simulink model "D53_LKAS_JLU_20200909_1512"  (R2018b)
settings: Solver=ode3  StartTime=0.0  StopTime=10.0  FixedStep=0.01  RelTol=1e-3  EnableMultiTasking=on
model workspace (MAT data in the model file):
  MCOS : class17 (value not decoded)
  MCOS : class17 (value not decoded)
  MCOS : class17 (value not decoded)
  MCOS : class17 (value not decoded)
  MCOS : class17 (value not decoded)
  MCOS : class17 (value not decoded)
  MCOS : class17 (value not decoded)
  MCOS : class17 (value not decoded)
  MCOS : class17 (value not decoded)
  MCOS : class17 (value not decoded)
  MCOS : class17 (value not decoded)
  MCOS : class17 (value not decoded)
  MCOS : class17 (value not decoded)
  MCOS : class17 (value not decoded)
  MCOS : class17 (value not decoded)
  MCOS : class17 (value not decoded)
  MCOS : class17 (value not decoded)
  MCOS : class17 (value not decoded)
  MCOS : class17 (value not decoded)
  MCOS : class17 (value not decoded)
  MCOS : class17 (value not decoded)
  MCOS : class17 (value not decoded)
  MCOS : class17 (value not decoded)
  MCOS : class17 (value not decoded)
  MCOS : class17 (value not decoded)
  MCOS : class17 (value not decoded)
  MCOS : class17 (value not decoded)
  MCOS : class17 (value not decoded)
  MCOS : class17 (value not decoded)
  MCOS : class17 (value not decoded)
  MCOS : class17 (value not decoded)
  MCOS : class17 (value not decoded)
  MCOS : class17 (value not decoded)
  MCOS : class17 (value not decoded)
  MCOS : class17 (value not decoded)
  MCOS : class17 (value not decoded)
  MCOS : class17 (value not decoded)
  MCOS : class17 (value not decoded)
  MCOS : class17 (value not decoded)
  MCOS : class17 (value not decoded)
  MCOS : class17 (value not decoded)
  MCOS : class17 (value not decoded)
  MCOS : class17 (value not decoded)
  MCOS : class17 (value not decoded)
  MCOS : class17 (value not decoded)
  MCOS : class17 (value not decoded)
  MCOS : class17 (value not decoded)
  MCOS : class17 (value not decoded)
  MCOS : class17 (value not decoded)
  MCOS : class17 (value not decoded)
  MCOS : class17 (value not decoded)
  MCOS : class17 (value not decoded)
  MCOS : class17 (value not decoded)
  MCOS : class17 (value not decoded)
  MCOS : class17 (value not decoded)
  MCOS : class17 (value not decoded)
  MCOS : class17 (value not decoded)
  MCOS : class17 (value not decoded)
  MCOS : class17 (value not decoded)
  MCOS : class17 (value not decoded)
  MCOS : class17 (value not decoded)
  MCOS : class17 (value not decoded)
  MCOS : class17 (value not decoded)
  MCOS : class17 (value not decoded)
  MCOS : class17 (value not decoded)
  MCOS : class17 (value not decoded)
  MCOS : class17 (value not decoded)
  MCOS : class17 (value not decoded)
  MCOS : class17 (value not decoded)
  MCOS : class17 (value not decoded)
  MCOS : class17 (value not decoded)
  MCOS : class17 (value not decoded)
  MCOS : class17 (value not decoded)
  MCOS : class17 (value not decoded)
  MCOS : class17 (value not decoded)
  MCOS : class17 (value not decoded)
  MCOS : class17 (value not decoded)
  MCOS : class17 (value not decoded)
  MCOS : class17 (value not decoded)
  MCOS : class17 (value not decoded)
  MCOS : class17 (value not decoded)
  MCOS : class17 (value not decoded)
  MCOS : class17 (value not decoded)
  MCOS : class17 (value not decoded)
  MCOS : class17 (value not decoded)
  MCOS : class17 (value not decoded)
  MCOS : class17 (value not decoded)
  MCOS : class17 (value not decoded)
  MCOS : class17 (value not decoded)
undefined symbols (not defined in the file): LKA_CarWidth, LKA_SampleTime, LKA_StrRatio_C, LKA_Veh2CamL_C, LKA_Veh2CamW_C, LKA_WhlBaseL_C, LL_CompSWA_C, LL_CrvtPrvwT_C, LL_DesDvt_C, LL_DvtComp_C, LL_DvtPrvwT_C, LL_DvtSpdDet_vDvtSpdMin_C, LL_HdAgExT_C, LL_HdAgPrvwT_C, LL_LAccMax_C, LL_LAccRMax_C, LL_LDW_EarliestWarnLine_C, LL_LDW_LatestWarnLine_C, LL_LDWS_SUPPRESS_HEADING, LL_LFClb_TFC_DiffCtlBalance, LL_LFClb_TFC_DiffCtrlMaxSWA, LL_LFClb_TFC_DiffCtrlRatio, LL_LFClb_TFC_facmGainLutGain1_C, LL_LFClb_TFC_facmGainLutGain2_C, LL_LFClb_TFC_facmIntegRatio, LL_LFClb_TFC_facmKlat_C, LL_LFClb_TFC_FfCtlRatio_C, LL_LFClb_TFC_phiIntegCtlMaxSWA_C, LL_LFClb_TFC_tiKlatPrvwT_C, LL_LFClb_TFC_vGainLutVehSpdLwr_C, LL_LFClb_TFC_vGainLutVehSpdUpr_C, LL_LKA_EarliestWarnLine_C, LL_LKA_LatestWarnLine_C, LL_LKAExPrcs_ExitC0Dvt, LL_LKAExPrcs_ExitC0Swt, LL_LKAExPrcs_tiExitTime1, LL_LKAExPrcs_tiExitTime2, LL_LKAExPrcs_tiExitTime3, LL_LKAS_OUT_OF_CONTROL_LAT_VEL, LL_LKAS_OUT_OF_CONTROL_TTLC, LL_LKASWASyn_M0, LL_LKASWASyn_M1, LL_LKASWASyn_M2, LL_LKASWASyn_M3K, LL_LKASWASyn_SWAaddMax, LL_LKASWASyn_T2, LL_LKASWASyn_tiTrqSwaRtTime, LL_LKASWASyn_tiTrqSwaTime, LL_LKASWASyn_TrqMax, LL_LKASWASyn_TrqSwaAddSwt, LL_LKASWASyn_TrqSwaRateDiff, LL_LSpdCompT_C, LL_lStpLngth_C, LL_MAX_DELAY_EPSSTAR_TIME, LL_MAX_DRIVER_TORQUE_DISABLE, LL_MAX_DRIVER_TORQUE_ENABLE, LL_MAX_LANE_WIDTH_DISABLE, LL_MAX_LANE_WIDTH_ENABLE, LL_MAX_LAT_ACC_DISABLE, LL_MAX_LAT_ACC_ENABLE ... (+30)
libraries: simulink x134, canmsglib x50, dspstat3 x3, simulink_extras x1
(part 5 of 17)

== system D53_LKAS_JLU_20200909_1512/SignalBusCreator/bsOriL0Info ==
  Bus Creator19 : BusCreator  Inputs=10
  CAN Pack : canmsglib/CAN Pack  CANdbFile=D:\LKAS\Documents\LKAS-Monitor.dbc  MsgList=Video_Lane_Left_A  MsgName=Video_Lane_Left_A  MsgIDType=Standard (11-bit identifier)  MsgIdentifier=1530  MsgLength=8  SignalInfo=C0_5FA$44$12$2$1$1$0$1.000000e-02$0$-2.048000e+01$2.047000e+01$#C1_5FA$50$10$2$1$1$0$9.765625e-04$0$-3.570000e-01$3.570000e-01$#C2_5FA$24$16$2$1$1$0$1.000000e-06$0$-3.276800e-02$3.276600e-02$#C3_5FA$8$16$2$1$1$0$4.000000e-09$0$-1.310720e-04$1.310680e-04$#Line_Type_5FA$59$3$2$2$1$0$1$0$0$7$#Quality_5FA$62$2$2$2$1$0$1$0$0$3$#  NSignals=6  StartBits=str2num('[int32(44);int32(50);int32(24);int32(8);int32(59);int32(62)]')  SignalSizes=str2num('[int32(12);int32(10);int32(16);int32(16);int32(3);int32(2)]')  ByteOrders=str2num('[int32(2);int32(2);int32(2);int32(2);int32(2);int32(2)]')  DataTypes=str2num('[int32(1);int32(1);int32(1);int32(1);int32(2);int32(2)]')  MultiplexTypes=str2num('[int32(1);int32(1);int32(1);int32(1);int32(1);int32(1)]')  MultiplexValues=str2num('[double(0);double(0);double(0);double(0);double(0);double(0)]')  Factors=str2num('[double(1.000000e-02);double(9.765625e-04);double(1.000000e-06);double(4.000000e-09);double(1);double(1)]')  Offsets=str2num('[double(0);double(0);double(0);double(0);double(0);double(0)]')  Minimums=str2num('[double(-2.048000e+01);double(-3.570000e-01);double(-3.276800e-02);double(-1.310720e-04);double(0);double(0)]')  Maximums=str2num('[double(2.047000e+01);double(3.570000e-01);double(3.276600e-02);double(1.310680e-04);double(7);double(3)]')  Remote=off  ApplyMinMax=off  BusOutput=off
      settings: SourceProductName=Simulink Real-Time  SourceProductBaseCode=XP  DataFormat=CANdb specified signals
  CAN Pack1 : canmsglib/CAN Pack  CANdbFile=D:\LKAS\Documents\LKAS-Monitor.dbc  MsgList=Video_Lane_Left_B  MsgName=Video_Lane_Left_B  MsgIDType=Standard (11-bit identifier)  MsgIdentifier=1532  MsgLength=4  SignalInfo=Line_Width_5FC$17$7$2$2$1$0$1.000000e-02$0$0$1.270000e+00$#Me_Line_Changed_5FC$16$1$2$2$1$0$1$0$0$1$#TLC_5FC$8$8$2$2$1$0$1.000000e-02$0$0$2.550000e+00$#View_Range_5FC$0$8$2$2$1$0$5.000000e-01$0$0$1.275000e+02$#  NSignals=4  StartBits=str2num('[int32(17);int32(16);int32(8);int32(0)]')  SignalSizes=str2num('[int32(7);int32(1);int32(8);int32(8)]')  ByteOrders=str2num('[int32(2);int32(2);int32(2);int32(2)]')  DataTypes=str2num('[int32(2);int32(2);int32(2);int32(2)]')  MultiplexTypes=str2num('[int32(1);int32(1);int32(1);int32(1)]')  MultiplexValues=str2num('[double(0);double(0);double(0);double(0)]')  Factors=str2num('[double(1.000000e-02);double(1);double(1.000000e-02);double(5.000000e-01)]')  Offsets=str2num('[double(0);double(0);double(0);double(0)]')  Minimums=str2num('[double(0);double(0);double(0);double(0)]')  Maximums=str2num('[double(1.270000e+00);double(1);double(2.550000e+00);double(1.275000e+02)]')  Remote=off  ApplyMinMax=off  BusOutput=off
      settings: SourceProductName=Simulink Real-Time  SourceProductBaseCode=XP  DataFormat=CANdb specified signals
  CAN Receive (CANRX) : S-Function  FunctionName=CAN_Rec_P  Parameters=uint8(Module-1),uint32(ID),uint8(Frameformat-1),uint8(Newflag),uint8(FIFO),double(sampletime)  SFunctionDeploymentMode=off  EnableBusSupport=off  mask(CAN_receive){Module=CAN_2, ID=1530, Frameformat=Standard (11-bit identifier), Newflag=off, FIFO=off, sampletime=0.05}
      mask prompts: Module "CAN Port:"; ID "CAN Frame ID:"; Frameformat "CAN Frame Format:"; FIFO "Overflow flag"
      mask init:
      | maskdisplay = canrecicon(Module,ID,Frameformat,Newflag,FIFO);
      | set_param(gcb, 'MaskDisplay', maskdisplay);
      mask TypeOptions Module: CAN_0 | CAN_1 | CAN_2 | CAN_3
      mask TypeOptions Frameformat: Standard (11-bit identifier) | Extended (29-bit identifier)
      mask Display: color('blue');text(0.98,0.9,'MPC5675K','horizontalAlignment','right');color('black');text(0.5,0.6,'FlexCAN_2 Receive','horizontalAlignment','center');text(0.5,0.35,'Standard ID:1530','horizontalAlignment','center');port_label('output',1,'CAN_Msg');
  CAN Receive (CANRX)1 : S-Function  FunctionName=CAN_Rec_P  Parameters=uint8(Module-1),uint32(ID),uint8(Frameformat-1),uint8(Newflag),uint8(FIFO),double(sampletime)  SFunctionDeploymentMode=off  EnableBusSupport=off  mask(CAN_receive){Module=CAN_2, ID=1532, Frameformat=Standard (11-bit identifier), Newflag=off, FIFO=off, sampletime=0.05}
      mask prompts: Module "CAN Port:"; ID "CAN Frame ID:"; Frameformat "CAN Frame Format:"; FIFO "Overflow flag"
      mask init:
      | maskdisplay = canrecicon(Module,ID,Frameformat,Newflag,FIFO);
      | set_param(gcb, 'MaskDisplay', maskdisplay);
      mask TypeOptions Module: CAN_0 | CAN_1 | CAN_2 | CAN_3
      mask TypeOptions Frameformat: Standard (11-bit identifier) | Extended (29-bit identifier)
      mask Display: color('blue');text(0.98,0.9,'MPC5675K','horizontalAlignment','right');color('black');text(0.5,0.6,'FlexCAN_2 Receive','horizontalAlignment','center');text(0.5,0.35,'Standard ID:1532','horizontalAlignment','center');port_label('output',1,'CAN_Msg');
  CAN Send1 : S-Function  FunctionName=CAN_Send_P  Parameters=uint8(CAN_Port-1),uint8(CAN_Priority-1),uint8(S_overflow_flag),uint8(S_timestamp),double(sampletime)  SFunctionDeploymentMode=off  EnableBusSupport=off  mask{CAN_Port=CAN_0, CAN_Priority=3, S_overflow_flag=off, S_timestamp=off, sampletime=0.05}
      mask prompts: CAN_Port "CAN Port:"; CAN_Priority "Priority:"; S_overflow_flag "Send overflow flag"; S_timestamp "Send time stamp"
      mask init:
      | maskdisplay = cansendicon(CAN_Port,CAN_Priority,S_overflow_flag,S_timestamp);
      | set_param(gcb, 'MaskDisplay', maskdisplay);
      mask TypeOptions CAN_Port: CAN_0 | CAN_1 | CAN_2 | CAN_3
      mask TypeOptions CAN_Priority: 0 | 1 | 2 | 3 | 4 | 5 | 6 | 7
      mask Display: color('blue');text(0.98,0.9,'MPC5675K','horizontalAlignment','right');color('black');text(0.5,0.6,'FlexCAN_0 Send','horizontalAlignment','center');text(0.5,0.35,'Priority:3','horizontalAlignment','center');port_label('input',1,'CAN_Msg');
  CAN Send2 : S-Function  FunctionName=CAN_Send_P  Parameters=uint8(CAN_Port-1),uint8(CAN_Priority-1),uint8(S_overflow_flag),uint8(S_timestamp),double(sampletime)  SFunctionDeploymentMode=off  EnableBusSupport=off  mask{CAN_Port=CAN_0, CAN_Priority=3, S_overflow_flag=off, S_timestamp=off, sampletime=0.05}
      mask prompts: CAN_Port "CAN Port:"; CAN_Priority "Priority:"; S_overflow_flag "Send overflow flag"; S_timestamp "Send time stamp"
      mask init:
      | maskdisplay = cansendicon(CAN_Port,CAN_Priority,S_overflow_flag,S_timestamp);
      | set_param(gcb, 'MaskDisplay', maskdisplay);
      mask TypeOptions CAN_Port: CAN_0 | CAN_1 | CAN_2 | CAN_3
      mask TypeOptions CAN_Priority: 0 | 1 | 2 | 3 | 4 | 5 | 6 | 7
      mask Display: color('blue');text(0.98,0.9,'MPC5675K','horizontalAlignment','right');color('black');text(0.5,0.6,'FlexCAN_0 Send','horizontalAlignment','center');text(0.5,0.35,'Priority:3','horizontalAlignment','center');port_label('input',1,'CAN_Msg');
  CAN Unpack1 : canmsglib/CAN Unpack  CANdbFile=D:\Work\02_LKA\LKAS\Documents\D53-SensorCAN.dbc  MsgList=Video_Lane_Left_B  MsgName=Video_Lane_Left_B  MsgIDType=Standard (11-bit identifier)  MsgIdentifier=1532  MsgLength=4  SignalInfo=Line_Width_5FC$17$7$2$2$1$0$1.000000e-02$0$0$1.270000e+00$#Me_Line_Changed_5FC$16$1$2$2$1$0$1$0$0$1$#TLC_5FC$8$8$2$2$1$0$1.000000e-02$0$0$2.550000e+00$#View_Range_5FC$0$8$2$2$1$0$5.000000e-01$0$0$1.275000e+02$#  NSignals=4  IDPort=off  TimestampPort=off  ErrorPort=off  RemotePort=off  LengthPort=off  StatusPort=off  StartBits=str2num('[int32(17);int32(16);int32(8);int32(0)]')  SignalSizes=str2num('[int32(7);int32(1);int32(8);int32(8)]')  ByteOrders=str2num('[int32(2);int32(2);int32(2);int32(2)]')  DataTypes=str2num('[int32(2);int32(2);int32(2);int32(2)]')  MultiplexTypes=str2num('[int32(1);int32(1);int32(1);int32(1)]')  MultiplexValues=str2num('[double(0);double(0);double(0);double(0)]')  Factors=str2num('[double(1.000000e-02);double(1);double(1.000000e-02);double(5.000000e-01)]')  Offsets=str2num('[double(0);double(0);double(0);double(0)]')  Minimums=str2num('[double(0);double(0);double(0);double(0)]')  Maximums=str2num('[double(1.270000e+00);double(1);double(2.550000e+00);double(1.275000e+02)]')  ApplyMinMax=off
      settings: SourceProductName=Simulink Real-Time  SourceProductBaseCode=XP  DataFormat=CANdb specified signals
  CAN Unpack13 : canmsglib/CAN Unpack  CANdbFile=D:\Work\02_LKA\LKAS\Documents\D53-SensorCAN.dbc  MsgList=Video_Lane_Left_A  MsgName=Video_Lane_Left_A  MsgIDType=Standard (11-bit identifier)  MsgIdentifier=1530  MsgLength=8  SignalInfo=C0_5FA$44$12$2$1$1$0$1.000000e-02$0$-2.048000e+01$2.047000e+01$#C1_5FA$50$10$2$1$1$0$9.765625e-04$0$-3.570000e-01$3.570000e-01$#C2_5FA$24$16$2$1$1$0$1.000000e-06$0$-3.276800e-02$3.276600e-02$#C3_5FA$8$16$2$1$1$0$4.000000e-09$0$-1.310720e-04$1.310680e-04$#Line_Type_5FA$59$3$2$2$1$0$1$0$0$7$#Quality_5FA$62$2$2$2$1$0$1$0$0$3$#  NSignals=6  IDPort=off  TimestampPort=off  ErrorPort=off  RemotePort=off  LengthPort=off  StatusPort=off  StartBits=str2num('[int32(44);int32(50);int32(24);int32(8);int32(59);int32(62)]')  SignalSizes=str2num('[int32(12);int32(10);int32(16);int32(16);int32(3);int32(2)]')  ByteOrders=str2num('[int32(2);int32(2);int32(2);int32(2);int32(2);int32(2)]')  DataTypes=str2num('[int32(1);int32(1);int32(1);int32(1);int32(2);int32(2)]')  MultiplexTypes=str2num('[int32(1);int32(1);int32(1);int32(1);int32(1);int32(1)]')  MultiplexValues=str2num('[double(0);double(0);double(0);double(0);double(0);double(0)]')  Factors=str2num('[double(1.000000e-02);double(9.765625e-04);double(1.000000e-06);double(4.000000e-09);double(1);double(1)]')  Offsets=str2num('[double(0);double(0);double(0);double(0);double(0);double(0)]')  Minimums=str2num('[double(-2.048000e+01);double(-3.570000e-01);double(-3.276800e-02);double(-1.310720e-04);double(0);double(0)]')  Maximums=str2num('[double(2.047000e+01);double(3.570000e-01);double(3.276600e-02);double(1.310680e-04);double(7);double(3)]')  ApplyMinMax=off
      settings: SourceProductName=Simulink Real-Time  SourceProductBaseCode=XP  DataFormat=CANdb specified signals
  Data Type Conversion{,1..3,5..6,9} (7 alike) : DataTypeConversion  OutDataTypeStr=single
  Data Type Conversion4 : DataTypeConversion  OutDataTypeStr=uint8
  Data Type Conversion7 : DataTypeConversion  OutDataTypeStr=uint8
  Data Type Conversion8 : DataTypeConversion  OutDataTypeStr=uint8
  Rate Transition{1..10} (10 alike) : RateTransition  Deterministic=off  OutPortSampleTime=0.01
  bsOriL0Info : Outport
  wires:
  Data Type Conversion1/1 -> Bus Creator19/3  "O_L0_C1"
  Data Type Conversion7/1 -> Bus Creator19/6  "O_L0_Type"
  CAN Unpack13/2 -> CAN Pack/2, Rate Transition9/1
  CAN Unpack1/1 -> CAN Pack1/1, Rate Transition4/1
  Data Type Conversion2/1 -> Bus Creator19/2  "O_L0_C2"
  CAN Unpack13/1 -> CAN Pack/1, Rate Transition10/1
  Data Type Conversion8/1 -> Bus Creator19/10  "O_L0_LC"
  Data Type Conversion/1 -> Bus Creator19/4  "O_L0_C0"
  Data Type Conversion4/1 -> Bus Creator19/5  "O_L0_Q"
  Data Type Conversion5/1 -> Bus Creator19/7  "O_L0_VR"
  Data Type Conversion3/1 -> Bus Creator19/1  "O_L0_C3"
  Data Type Conversion9/1 -> Bus Creator19/8  "O_L0_TLC"
  CAN Unpack13/5 -> CAN Pack/5, Rate Transition6/1
  CAN Unpack1/2 -> CAN Pack1/2, Rate Transition3/1
  CAN Unpack1/4 -> CAN Pack1/4, Rate Transition1/1
  Data Type Conversion6/1 -> Bus Creator19/9  "O_L0_W"
  CAN Unpack13/3 -> CAN Pack/3, Rate Transition8/1
  CAN Unpack1/3 -> CAN Pack1/3, Rate Transition2/1
  CAN Unpack13/6 -> CAN Pack/6, Rate Transition5/1
  CAN Unpack13/4 -> CAN Pack/4, Rate Transition7/1
  Bus Creator19/1 -> bsOriL0Info/1  "bsOriL0Info"
  CAN Receive (CANRX)/1 -> CAN Unpack13/1
  CAN Receive (CANRX)1/1 -> CAN Unpack1/1
  Rate Transition1/1 -> Data Type Conversion5/1
  Rate Transition2/1 -> Data Type Conversion9/1
  Rate Transition3/1 -> Data Type Conversion8/1
  Rate Transition4/1 -> Data Type Conversion6/1
  Rate Transition5/1 -> Data Type Conversion4/1
  Rate Transition6/1 -> Data Type Conversion7/1
  Rate Transition7/1 -> Data Type Conversion3/1
  Rate Transition8/1 -> Data Type Conversion2/1
  Rate Transition10/1 -> Data Type Conversion/1
  Rate Transition9/1 -> Data Type Conversion1/1
  CAN Pack/1 -> CAN Send2/1
  CAN Pack1/1 -> CAN Send1/1

== system D53_LKAS_JLU_20200909_1512/SignalBusCreator/bsOriL1Info ==
  Bus Creator20 : BusCreator  Inputs=10
  CAN Receive (CANRX) : S-Function  FunctionName=CAN_Rec_P  Parameters=uint8(Module-1),uint32(ID),uint8(Frameformat-1),uint8(Newflag),uint8(FIFO),double(sampletime)  SFunctionDeploymentMode=off  EnableBusSupport=off  mask(CAN_receive){Module=CAN_2, ID=1531, Frameformat=Standard (11-bit identifier), Newflag=off, FIFO=off, sampletime=0.05}
      mask prompts: Module "CAN Port:"; ID "CAN Frame ID:"; Frameformat "CAN Frame Format:"; FIFO "Overflow flag"
      mask init:
      | maskdisplay = canrecicon(Module,ID,Frameformat,Newflag,FIFO);
      | set_param(gcb, 'MaskDisplay', maskdisplay);
      mask TypeOptions Module: CAN_0 | CAN_1 | CAN_2 | CAN_3
      mask TypeOptions Frameformat: Standard (11-bit identifier) | Extended (29-bit identifier)
      mask Display: color('blue');text(0.98,0.9,'MPC5675K','horizontalAlignment','right');color('black');text(0.5,0.6,'FlexCAN_2 Receive','horizontalAlignment','center');text(0.5,0.35,'Standard ID:1531','horizontalAlignment','center');port_label('output',1,'CAN_Msg');
  CAN Receive (CANRX)1 : S-Function  FunctionName=CAN_Rec_P  Parameters=uint8(Module-1),uint32(ID),uint8(Frameformat-1),uint8(Newflag),uint8(FIFO),double(sampletime)  SFunctionDeploymentMode=off  EnableBusSupport=off  mask(CAN_receive){Module=CAN_2, ID=1523, Frameformat=Standard (11-bit identifier), Newflag=off, FIFO=off, sampletime=0.05}
      mask prompts: Module "CAN Port:"; ID "CAN Frame ID:"; Frameformat "CAN Frame Format:"; FIFO "Overflow flag"
      mask init:
      | maskdisplay = canrecicon(Module,ID,Frameformat,Newflag,FIFO);
      | set_param(gcb, 'MaskDisplay', maskdisplay);
      mask TypeOptions Module: CAN_0 | CAN_1 | CAN_2 | CAN_3
      mask TypeOptions Frameformat: Standard (11-bit identifier) | Extended (29-bit identifier)
      mask Display: color('blue');text(0.98,0.9,'MPC5675K','horizontalAlignment','right');color('black');text(0.5,0.6,'FlexCAN_2 Receive','horizontalAlignment','center');text(0.5,0.35,'Standard ID:1523','horizontalAlignment','center');port_label('output',1,'CAN_Msg');
  CAN Unpack1 : canmsglib/CAN Unpack  CANdbFile=D:\Work\02_LKA\LKAS\Documents\D53-SensorCAN.dbc  MsgList=Video_Lane_Next_Left_B  MsgName=Video_Lane_Next_Left_B  MsgIDType=Standard (11-bit identifier)  MsgIdentifier=1523  MsgLength=4  SignalInfo=Line_Width_5F3$17$7$2$2$1$0$1.000000e-02$0$0$1.270000e+00$#Me_Line_Changed_5F3$16$1$2$2$1$0$1$0$0$1$#TLC_5F3$8$8$2$2$1$0$1.000000e-02$0$0$2.550000e+00$#View_Range_5F3$0$8$2$2$1$0$5.000000e-01$0$0$1.275000e+02$#  NSignals=4  IDPort=off  TimestampPort=off  ErrorPort=off  RemotePort=off  LengthPort=off  StatusPort=off  StartBits=str2num('[int32(17);int32(16);int32(8);int32(0)]')  SignalSizes=str2num('[int32(7);int32(1);int32(8);int32(8)]')  ByteOrders=str2num('[int32(2);int32(2);int32(2);int32(2)]')  DataTypes=str2num('[int32(2);int32(2);int32(2);int32(2)]')  MultiplexTypes=str2num('[int32(1);int32(1);int32(1);int32(1)]')  MultiplexValues=str2num('[double(0);double(0);double(0);double(0)]')  Factors=str2num('[double(1.000000e-02);double(1);double(1.000000e-02);double(5.000000e-01)]')  Offsets=str2num('[double(0);double(0);double(0);double(0)]')  Minimums=str2num('[double(0);double(0);double(0);double(0)]')  Maximums=str2num('[double(1.270000e+00);double(1);double(2.550000e+00);double(1.275000e+02)]')  ApplyMinMax=off
      settings: SourceProductName=Simulink Real-Time  SourceProductBaseCode=XP  DataFormat=CANdb specified signals
  CAN Unpack13 : canmsglib/CAN Unpack  CANdbFile=D:\Work\02_LKA\LKAS\Documents\D53-SensorCAN.dbc  MsgList=Video_Lane_Next_Left_A  MsgName=Video_Lane_Next_Left_A  MsgIDType=Standard (11-bit identifier)  MsgIdentifier=1531  MsgLength=8  SignalInfo=C0_5FB$44$12$2$1$1$0$1.000000e-02$0$-2.048000e+01$2.047000e+01$#C1_5FB$50$10$2$1$1$0$9.765625e-04$0$-3.570000e-01$3.570000e-01$#C2_5FB$24$16$2$1$1$0$1.000000e-06$0$-3.276800e-02$3.276600e-02$#C3_5FB$8$16$2$1$1$0$4.000000e-09$0$-1.310720e-04$1.310680e-04$#Line_Type_5FB$59$3$2$2$1$0$1$0$0$7$#Quality_5FB$62$2$2$2$1$0$1$0$0$3$#  NSignals=6  IDPort=off  TimestampPort=off  ErrorPort=off  RemotePort=off  LengthPort=off  StatusPort=off  StartBits=str2num('[int32(44);int32(50);int32(24);int32(8);int32(59);int32(62)]')  SignalSizes=str2num('[int32(12);int32(10);int32(16);int32(16);int32(3);int32(2)]')  ByteOrders=str2num('[int32(2);int32(2);int32(2);int32(2);int32(2);int32(2)]')  DataTypes=str2num('[int32(1);int32(1);int32(1);int32(1);int32(2);int32(2)]')  MultiplexTypes=str2num('[int32(1);int32(1);int32(1);int32(1);int32(1);int32(1)]')  MultiplexValues=str2num('[double(0);double(0);double(0);double(0);double(0);double(0)]')  Factors=str2num('[double(1.000000e-02);double(9.765625e-04);double(1.000000e-06);double(4.000000e-09);double(1);double(1)]')  Offsets=str2num('[double(0);double(0);double(0);double(0);double(0);double(0)]')  Minimums=str2num('[double(-2.048000e+01);double(-3.570000e-01);double(-3.276800e-02);double(-1.310720e-04);double(0);double(0)]')  Maximums=str2num('[double(2.047000e+01);double(3.570000e-01);double(3.276600e-02);double(1.310680e-04);double(7);double(3)]')  ApplyMinMax=off
      settings: SourceProductName=Simulink Real-Time  SourceProductBaseCode=XP  DataFormat=CANdb specified signals
  Data Type Conversion{,1..3,5..6,9} (7 alike) : DataTypeConversion  OutDataTypeStr=single
  Data Type Conversion4 : DataTypeConversion  OutDataTypeStr=uint8
  Data Type Conversion7 : DataTypeConversion  OutDataTypeStr=uint8
  Data Type Conversion8 : DataTypeConversion  OutDataTypeStr=uint8
  Rate Transition{1..10} (10 alike) : RateTransition  Deterministic=off  OutPortSampleTime=0.01
  bsOriL1Info : Outport
  wires:
  CAN Receive (CANRX)/1 -> CAN Unpack13/1
  Data Type Conversion/1 -> Bus Creator20/4  "O_L1_C0"
  CAN Unpack13/4 -> Rate Transition7/1
  CAN Unpack13/5 -> Rate Transition6/1
  Data Type Conversion6/1 -> Bus Creator20/9  "O_L1_W"
  CAN Unpack13/2 -> Rate Transition9/1
  CAN Unpack1/4 -> Rate Transition1/1
  Data Type Conversion4/1 -> Bus Creator20/5  "O_L1_Q"
  CAN Unpack1/2 -> Rate Transition3/1
  CAN Unpack13/6 -> Rate Transition5/1
  CAN Unpack13/1 -> Rate Transition10/1
  CAN Unpack1/1 -> Rate Transition4/1
  CAN Unpack1/3 -> Rate Transition2/1
  CAN Unpack13/3 -> Rate Transition8/1
  Data Type Conversion9/1 -> Bus Creator20/8  "O_L1_TLC"
  Data Type Conversion7/1 -> Bus Creator20/6  "O_L1_Type"
  Bus Creator20/1 -> bsOriL1Info/1  "bsOriL1Info"
  Data Type Conversion5/1 -> Bus Creator20/7  "O_L1_VR"
  Data Type Conversion3/1 -> Bus Creator20/1  "O_L1_C3"
  Data Type Conversion8/1 -> Bus Creator20/10  "O_L1_LC"
  Data Type Conversion1/1 -> Bus Creator20/3  "O_L1_C1"
  Data Type Conversion2/1 -> Bus Creator20/2  "O_L1_C2"
  CAN Receive (CANRX)1/1 -> CAN Unpack1/1
  Rate Transition1/1 -> Data Type Conversion5/1
  Rate Transition2/1 -> Data Type Conversion9/1
  Rate Transition3/1 -> Data Type Conversion8/1
  Rate Transition4/1 -> Data Type Conversion6/1
  Rate Transition5/1 -> Data Type Conversion4/1
  Rate Transition6/1 -> Data Type Conversion7/1
  Rate Transition7/1 -> Data Type Conversion3/1
  Rate Transition8/1 -> Data Type Conversion2/1
  Rate Transition9/1 -> Data Type Conversion1/1
  Rate Transition10/1 -> Data Type Conversion/1

== system D53_LKAS_JLU_20200909_1512/SignalBusCreator/bsOriLaneInfo ==
  Bus Creator18 : BusCreator  Inputs=3
  CAN Recv : S-Function  FunctionName=CAN_Rec_P  Parameters=uint8(Module-1),uint32(ID),uint8(Frameformat-1),uint8(Newflag),uint8(FIFO),double(sampletime)  SFunctionDeploymentMode=off  EnableBusSupport=off  mask(CAN_receive){Module=CAN_2, ID=1110, Frameformat=Standard (11-bit identifier), Newflag=off, FIFO=off, sampletime=0.05}
      mask prompts: Module "CAN Port:"; ID "CAN Frame ID:"; Frameformat "CAN Frame Format:"; FIFO "Overflow flag"
      mask init:
      | maskdisplay = canrecicon(Module,ID,Frameformat,Newflag,FIFO);
      | set_param(gcb, 'MaskDisplay', maskdisplay);
      mask TypeOptions Module: CAN_0 | CAN_1 | CAN_2 | CAN_3
      mask TypeOptions Frameformat: Standard (11-bit identifier) | Extended (29-bit identifier)
      mask Display: color('blue');text(0.98,0.9,'MPC5675K','horizontalAlignment','right');color('black');text(0.5,0.6,'FlexCAN_2 Receive','horizontalAlignment','center');text(0.5,0.35,'Standard ID:1110','horizontalAlignment','center');port_label('output',1,'CAN_Msg');
  CAN Unpack : canmsglib/CAN Unpack  CANdbFile=D:\Work\02_LKA\LKAS\Documents\D53-SensorCAN.dbc  MsgList=Video_Lane_Header  MsgName=Video_Lane_Header  MsgIDType=Standard (11-bit identifier)  MsgIdentifier=1110  MsgLength=1  SignalInfo=Construction_Area$6$1$2$2$1$0$1$0$0$1$#LaneModuleValid$7$1$2$2$1$0$1$0$0$1$#Road_Type$4$2$2$2$1$0$1$0$0$3$#  NSignals=3  IDPort=off  TimestampPort=off  ErrorPort=off  RemotePort=off  LengthPort=off  StatusPort=off  StartBits=str2num('[int32(6);int32(7);int32(4)]')  SignalSizes=str2num('[int32(1);int32(1);int32(2)]')  ByteOrders=str2num('[int32(2);int32(2);int32(2)]')  DataTypes=str2num('[int32(2);int32(2);int32(2)]')  MultiplexTypes=str2num('[int32(1);int32(1);int32(1)]')  MultiplexValues=str2num('[double(0);double(0);double(0)]')  Factors=str2num('[double(1);double(1);double(1)]')  Offsets=str2num('[double(0);double(0);double(0)]')  Minimums=str2num('[double(0);double(0);double(0)]')  Maximums=str2num('[double(1);double(1);double(3)]')  ApplyMinMax=off
      settings: SourceProductName=Simulink Real-Time  SourceProductBaseCode=XP  DataFormat=CANdb specified signals
  Data Type Conversion : DataTypeConversion  OutDataTypeStr=uint8
  Data Type Conversion1 : DataTypeConversion  OutDataTypeStr=uint8
  Data Type Conversion2 : DataTypeConversion  OutDataTypeStr=uint8
  Rate Transition1 : RateTransition  Deterministic=off  OutPortSampleTime=0.01
  Rate Transition2 : RateTransition  Deterministic=off  OutPortSampleTime=0.01
  Rate Transition3 : RateTransition  Deterministic=off  OutPortSampleTime=0.01
  bsOriLaneInfo : Outport
  wires:
  CAN Unpack/3 -> Rate Transition3/1  "O_Lane_RoadType"
  CAN Unpack/2 -> Rate Transition2/1  "O_Lane_Valid"
  CAN Recv/1 -> CAN Unpack/1
  CAN Unpack/1 -> Rate Transition1/1  "O_Lane_ConsArea"
  Bus Creator18/1 -> bsOriLaneInfo/1  "bsOriLaneInfo"
  Data Type Conversion/1 -> Bus Creator18/2  "O_Lane_ConsArea"
  Data Type Conversion1/1 -> Bus Creator18/1  "O_Lane_Valid"
  Data Type Conversion2/1 -> Bus Creator18/3  "O_Lane_RoadType"
  Rate Transition1/1 -> Data Type Conversion/1
  Rate Transition2/1 -> Data Type Conversion1/1
  Rate Transition3/1 -> Data Type Conversion2/1

== system D53_LKAS_JLU_20200909_1512/SignalBusCreator/bsOriR0Info ==
  Bus Creator21 : BusCreator  Inputs=10
  CAN Pack : canmsglib/CAN Pack  CANdbFile=D:\LKAS\Documents\LKAS-Monitor.dbc  MsgList=Video_Lane_Right_B  MsgName=Video_Lane_Right_B  MsgIDType=Standard (11-bit identifier)  MsgIdentifier=1535  MsgLength=4  SignalInfo=Line_Width_5FF$17$7$2$2$1$0$1.000000e-02$0$0$1.270000e+00$#Me_Line_Changed_5FF$16$1$2$2$1$0$1$0$0$1$#TLC_5FF$8$8$2$2$1$0$1.000000e-02$0$0$2.550000e+00$#View_Range_5FF$0$8$2$2$1$0$5.000000e-01$0$0$1.275000e+02$#  NSignals=4  StartBits=str2num('[int32(17);int32(16);int32(8);int32(0)]')  SignalSizes=str2num('[int32(7);int32(1);int32(8);int32(8)]')  ByteOrders=str2num('[int32(2);int32(2);int32(2);int32(2)]')  DataTypes=str2num('[int32(2);int32(2);int32(2);int32(2)]')  MultiplexTypes=str2num('[int32(1);int32(1);int32(1);int32(1)]')  MultiplexValues=str2num('[double(0);double(0);double(0);double(0)]')  Factors=str2num('[double(1.000000e-02);double(1);double(1.000000e-02);double(5.000000e-01)]')  Offsets=str2num('[double(0);double(0);double(0);double(0)]')  Minimums=str2num('[double(0);double(0);double(0);double(0)]')  Maximums=str2num('[double(1.270000e+00);double(1);double(2.550000e+00);double(1.275000e+02)]')  Remote=off  ApplyMinMax=off  BusOutput=off
      settings: SourceProductName=Simulink Real-Time  SourceProductBaseCode=XP  DataFormat=CANdb specified signals
  CAN Pack1 : canmsglib/CAN Pack  CANdbFile=D:\LKAS\Documents\LKAS-Monitor.dbc  MsgList=Video_Lane_Right_A  MsgName=Video_Lane_Right_A  MsgIDType=Standard (11-bit identifier)  MsgIdentifier=1533  MsgLength=8  SignalInfo=C0_5FD$44$12$2$1$1$0$1.000000e-02$0$-2.048000e+01$2.047000e+01$#C1_5FD$50$10$2$1$1$0$9.765625e-04$0$-3.570000e-01$3.570000e-01$#C2_5FD$24$16$2$1$1$0$1.000000e-06$0$-3.276800e-02$3.276600e-02$#C3_5FD$8$16$2$1$1$0$4.000000e-09$0$-1.310720e-04$1.310680e-04$#Line_Type_5FD$59$3$2$2$1$0$1$0$0$7$#Quality_5FD$62$2$2$2$1$0$1$0$0$3$#  NSignals=6  StartBits=str2num('[int32(44);int32(50);int32(24);int32(8);int32(59);int32(62)]')  SignalSizes=str2num('[int32(12);int32(10);int32(16);int32(16);int32(3);int32(2)]')  ByteOrders=str2num('[int32(2);int32(2);int32(2);int32(2);int32(2);int32(2)]')  DataTypes=str2num('[int32(1);int32(1);int32(1);int32(1);int32(2);int32(2)]')  MultiplexTypes=str2num('[int32(1);int32(1);int32(1);int32(1);int32(1);int32(1)]')  MultiplexValues=str2num('[double(0);double(0);double(0);double(0);double(0);double(0)]')  Factors=str2num('[double(1.000000e-02);double(9.765625e-04);double(1.000000e-06);double(4.000000e-09);double(1);double(1)]')  Offsets=str2num('[double(0);double(0);double(0);double(0);double(0);double(0)]')  Minimums=str2num('[double(-2.048000e+01);double(-3.570000e-01);double(-3.276800e-02);double(-1.310720e-04);double(0);double(0)]')  Maximums=str2num('[double(2.047000e+01);double(3.570000e-01);double(3.276600e-02);double(1.310680e-04);double(7);double(3)]')  Remote=off  ApplyMinMax=off  BusOutput=off
      settings: SourceProductName=Simulink Real-Time  SourceProductBaseCode=XP  DataFormat=CANdb specified signals
  CAN Receive (CANRX) : S-Function  FunctionName=CAN_Rec_P  Parameters=uint8(Module-1),uint32(ID),uint8(Frameformat-1),uint8(Newflag),uint8(FIFO),double(sampletime)  SFunctionDeploymentMode=off  EnableBusSupport=off  mask(CAN_receive){Module=CAN_2, ID=1533, Frameformat=Standard (11-bit identifier), Newflag=off, FIFO=off, sampletime=0.05}
      mask prompts: Module "CAN Port:"; ID "CAN Frame ID:"; Frameformat "CAN Frame Format:"; FIFO "Overflow flag"
      mask init:
      | maskdisplay = canrecicon(Module,ID,Frameformat,Newflag,FIFO);
      | set_param(gcb, 'MaskDisplay', maskdisplay);
      mask TypeOptions Module: CAN_0 | CAN_1 | CAN_2 | CAN_3
      mask TypeOptions Frameformat: Standard (11-bit identifier) | Extended (29-bit identifier)
      mask Display: color('blue');text(0.98,0.9,'MPC5675K','horizontalAlignment','right');color('black');text(0.5,0.6,'FlexCAN_2 Receive','horizontalAlignment','center');text(0.5,0.35,'Standard ID:1533','horizontalAlignment','center');port_label('output',1,'CAN_Msg');
  CAN Receive (CANRX)1 : S-Function  FunctionName=CAN_Rec_P  Parameters=uint8(Module-1),uint32(ID),uint8(Frameformat-1),uint8(Newflag),uint8(FIFO),double(sampletime)  SFunctionDeploymentMode=off  EnableBusSupport=off  mask(CAN_receive){Module=CAN_2, ID=1535, Frameformat=Standard (11-bit identifier), Newflag=off, FIFO=off, sampletime=0.05}
      mask prompts: Module "CAN Port:"; ID "CAN Frame ID:"; Frameformat "CAN Frame Format:"; FIFO "Overflow flag"
      mask init:
      | maskdisplay = canrecicon(Module,ID,Frameformat,Newflag,FIFO);
      | set_param(gcb, 'MaskDisplay', maskdisplay);
      mask TypeOptions Module: CAN_0 | CAN_1 | CAN_2 | CAN_3
      mask TypeOptions Frameformat: Standard (11-bit identifier) | Extended (29-bit identifier)
      mask Display: color('blue');text(0.98,0.9,'MPC5675K','horizontalAlignment','right');color('black');text(0.5,0.6,'FlexCAN_2 Receive','horizontalAlignment','center');text(0.5,0.35,'Standard ID:1535','horizontalAlignment','center');port_label('output',1,'CAN_Msg');
  CAN Send2 : S-Function  FunctionName=CAN_Send_P  Parameters=uint8(CAN_Port-1),uint8(CAN_Priority-1),uint8(S_overflow_flag),uint8(S_timestamp),double(sampletime)  SFunctionDeploymentMode=off  EnableBusSupport=off  mask{CAN_Port=CAN_0, CAN_Priority=3, S_overflow_flag=off, S_timestamp=off, sampletime=0.05}
      mask prompts: CAN_Port "CAN Port:"; CAN_Priority "Priority:"; S_overflow_flag "Send overflow flag"; S_timestamp "Send time stamp"
      mask init:
      | maskdisplay = cansendicon(CAN_Port,CAN_Priority,S_overflow_flag,S_timestamp);
      | set_param(gcb, 'MaskDisplay', maskdisplay);
      mask TypeOptions CAN_Port: CAN_0 | CAN_1 | CAN_2 | CAN_3
      mask TypeOptions CAN_Priority: 0 | 1 | 2 | 3 | 4 | 5 | 6 | 7
      mask Display: color('blue');text(0.98,0.9,'MPC5675K','horizontalAlignment','right');color('black');text(0.5,0.6,'FlexCAN_0 Send','horizontalAlignment','center');text(0.5,0.35,'Priority:3','horizontalAlignment','center');port_label('input',1,'CAN_Msg');
  CAN Send3 : S-Function  FunctionName=CAN_Send_P  Parameters=uint8(CAN_Port-1),uint8(CAN_Priority-1),uint8(S_overflow_flag),uint8(S_timestamp),double(sampletime)  SFunctionDeploymentMode=off  EnableBusSupport=off  mask{CAN_Port=CAN_0, CAN_Priority=3, S_overflow_flag=off, S_timestamp=off, sampletime=0.05}
      mask prompts: CAN_Port "CAN Port:"; CAN_Priority "Priority:"; S_overflow_flag "Send overflow flag"; S_timestamp "Send time stamp"
      mask init:
      | maskdisplay = cansendicon(CAN_Port,CAN_Priority,S_overflow_flag,S_timestamp);
      | set_param(gcb, 'MaskDisplay', maskdisplay);
      mask TypeOptions CAN_Port: CAN_0 | CAN_1 | CAN_2 | CAN_3
      mask TypeOptions CAN_Priority: 0 | 1 | 2 | 3 | 4 | 5 | 6 | 7
      mask Display: color('blue');text(0.98,0.9,'MPC5675K','horizontalAlignment','right');color('black');text(0.5,0.6,'FlexCAN_0 Send','horizontalAlignment','center');text(0.5,0.35,'Priority:3','horizontalAlignment','center');port_label('input',1,'CAN_Msg');
  CAN Unpack1 : canmsglib/CAN Unpack  CANdbFile=D:\Work\02_LKA\LKAS\Documents\D53-SensorCAN.dbc  MsgList=Video_Lane_Right_B  MsgName=Video_Lane_Right_B  MsgIDType=Standard (11-bit identifier)  MsgIdentifier=1535  MsgLength=4  SignalInfo=Line_Width_5FF$17$7$2$2$1$0$1.000000e-02$0$0$1.270000e+00$#Me_Line_Changed_5FF$16$1$2$2$1$0$1$0$0$1$#TLC_5FF$8$8$2$2$1$0$1.000000e-02$0$0$2.550000e+00$#View_Range_5FF$0$8$2$2$1$0$5.000000e-01$0$0$1.275000e+02$#  NSignals=4  IDPort=off  TimestampPort=off  ErrorPort=off  RemotePort=off  LengthPort=off  StatusPort=off  StartBits=str2num('[int32(17);int32(16);int32(8);int32(0)]')  SignalSizes=str2num('[int32(7);int32(1);int32(8);int32(8)]')  ByteOrders=str2num('[int32(2);int32(2);int32(2);int32(2)]')  DataTypes=str2num('[int32(2);int32(2);int32(2);int32(2)]')  MultiplexTypes=str2num('[int32(1);int32(1);int32(1);int32(1)]')  MultiplexValues=str2num('[double(0);double(0);double(0);double(0)]')  Factors=str2num('[double(1.000000e-02);double(1);double(1.000000e-02);double(5.000000e-01)]')  Offsets=str2num('[double(0);double(0);double(0);double(0)]')  Minimums=str2num('[double(0);double(0);double(0);double(0)]')  Maximums=str2num('[double(1.270000e+00);double(1);double(2.550000e+00);double(1.275000e+02)]')  ApplyMinMax=off
      settings: SourceProductName=Simulink Real-Time  SourceProductBaseCode=XP  DataFormat=CANdb specified signals
  CAN Unpack14 : canmsglib/CAN Unpack  CANdbFile=D:\Work\02_LKA\LKAS\Documents\D53-SensorCAN.dbc  MsgList=Video_Lane_Right_A  MsgName=Video_Lane_Right_A  MsgIDType=Standard (11-bit identifier)  MsgIdentifier=1533  MsgLength=8  SignalInfo=C0_5FD$44$12$2$1$1$0$1.000000e-02$0$-2.048000e+01$2.047000e+01$#C1_5FD$50$10$2$1$1$0$9.765625e-04$0$-3.570000e-01$3.570000e-01$#C2_5FD$24$16$2$1$1$0$1.000000e-06$0$-3.276800e-02$3.276600e-02$#C3_5FD$8$16$2$1$1$0$4.000000e-09$0$-1.310720e-04$1.310680e-04$#Line_Type_5FD$59$3$2$2$1$0$1$0$0$7$#Quality_5FD$62$2$2$2$1$0$1$0$0$3$#  NSignals=6  IDPort=off  TimestampPort=off  ErrorPort=off  RemotePort=off  LengthPort=off  StatusPort=off  StartBits=str2num('[int32(44);int32(50);int32(24);int32(8);int32(59);int32(62)]')  SignalSizes=str2num('[int32(12);int32(10);int32(16);int32(16);int32(3);int32(2)]')  ByteOrders=str2num('[int32(2);int32(2);int32(2);int32(2);int32(2);int32(2)]')  DataTypes=str2num('[int32(1);int32(1);int32(1);int32(1);int32(2);int32(2)]')  MultiplexTypes=str2num('[int32(1);int32(1);int32(1);int32(1);int32(1);int32(1)]')  MultiplexValues=str2num('[double(0);double(0);double(0);double(0);double(0);double(0)]')  Factors=str2num('[double(1.000000e-02);double(9.765625e-04);double(1.000000e-06);double(4.000000e-09);double(1);double(1)]')  Offsets=str2num('[double(0);double(0);double(0);double(0);double(0);double(0)]')  Minimums=str2num('[double(-2.048000e+01);double(-3.570000e-01);double(-3.276800e-02);double(-1.310720e-04);double(0);double(0)]')  Maximums=str2num('[double(2.047000e+01);double(3.570000e-01);double(3.276600e-02);double(1.310680e-04);double(7);double(3)]')  ApplyMinMax=off
      settings: SourceProductName=Simulink Real-Time  SourceProductBaseCode=XP  DataFormat=CANdb specified signals
  Data Type Conversion{1..4,6..7,10} (7 alike) : DataTypeConversion  OutDataTypeStr=single
  Data Type Conversion5 : DataTypeConversion  OutDataTypeStr=uint8
  Data Type Conversion8 : DataTypeConversion  OutDataTypeStr=uint8
  Data Type Conversion9 : DataTypeConversion  OutDataTypeStr=uint8
  Rate Transition{1..10} (10 alike) : RateTransition  Deterministic=off  OutPortSampleTime=0.01
  bsOriR0Info : Outport
  wires:
  Data Type Conversion4/1 -> Bus Creator21/4  "O_R0_C0"
  CAN Unpack1/4 -> CAN Pack/4, Rate Transition1/1
  Data Type Conversion1/1 -> Bus Creator21/3  "O_R0_C1"
  Data Type Conversion7/1 -> Bus Creator21/9  "O_R0_W"
  Data Type Conversion10/1 -> Bus Creator21/8  "O_R0_TLC"
  CAN Receive (CANRX)1/1 -> CAN Unpack1/1
  CAN Unpack1/2 -> CAN Pack/2, Rate Transition3/1
  Data Type Conversion9/1 -> Bus Creator21/10  "O_R0_LC"
  Data Type Conversion6/1 -> Bus Creator21/7  "O_R0_VR"
  CAN Unpack14/1 -> CAN Pack1/1, Rate Transition10/1
  Data Type Conversion2/1 -> Bus Creator21/2  "O_R0_C2"
  CAN Unpack14/3 -> CAN Pack1/3, Rate Transition8/1
  CAN Unpack1/3 -> CAN Pack/3, Rate Transition2/1
  Data Type Conversion8/1 -> Bus Creator21/6  "O_R0_Type"
  Data Type Conversion3/1 -> Bus Creator21/1  "O_R0_C3"
  CAN Unpack14/6 -> CAN Pack1/6, Rate Transition5/1
  CAN Unpack14/2 -> CAN Pack1/2, Rate Transition9/1
  CAN Unpack14/4 -> CAN Pack1/4, Rate Transition7/1
  CAN Unpack14/5 -> CAN Pack1/5, Rate Transition6/1
  Data Type Conversion5/1 -> Bus Creator21/5  "O_R0_Q"
  CAN Unpack1/1 -> CAN Pack/1, Rate Transition4/1
  Bus Creator21/1 -> bsOriR0Info/1  "bsOriR0Info"
  CAN Receive (CANRX)/1 -> CAN Unpack14/1
  Rate Transition1/1 -> Data Type Conversion6/1
  Rate Transition2/1 -> Data Type Conversion10/1
  Rate Transition3/1 -> Data Type Conversion9/1
  Rate Transition4/1 -> Data Type Conversion7/1
  Rate Transition5/1 -> Data Type Conversion5/1
  Rate Transition6/1 -> Data Type Conversion8/1
  Rate Transition7/1 -> Data Type Conversion3/1
  Rate Transition9/1 -> Data Type Conversion1/1
  Rate Transition8/1 -> Data Type Conversion2/1
  Rate Transition10/1 -> Data Type Conversion4/1
  CAN Pack/1 -> CAN Send3/1
  CAN Pack1/1 -> CAN Send2/1

== system D53_LKAS_JLU_20200909_1512/SignalBusCreator/bsOriR1Info ==
  Bus Creator22 : BusCreator  Inputs=10
  CAN Receive (CANRX) : S-Function  FunctionName=CAN_Rec_P  Parameters=uint8(Module-1),uint32(ID),uint8(Frameformat-1),uint8(Newflag),uint8(FIFO),double(sampletime)  SFunctionDeploymentMode=off  EnableBusSupport=off  mask(CAN_receive){Module=CAN_2, ID=1534, Frameformat=Standard (11-bit identifier), Newflag=off, FIFO=off, sampletime=0.05}
      mask prompts: Module "CAN Port:"; ID "CAN Frame ID:"; Frameformat "CAN Frame Format:"; FIFO "Overflow flag"
      mask init:
      | maskdisplay = canrecicon(Module,ID,Frameformat,Newflag,FIFO);
      | set_param(gcb, 'MaskDisplay', maskdisplay);
      mask TypeOptions Module: CAN_0 | CAN_1 | CAN_2 | CAN_3
      mask TypeOptions Frameformat: Standard (11-bit identifier) | Extended (29-bit identifier)
      mask Display: color('blue');text(0.98,0.9,'MPC5675K','horizontalAlignment','right');color('black');text(0.5,0.6,'FlexCAN_2 Receive','horizontalAlignment','center');text(0.5,0.35,'Standard ID:1534','horizontalAlignment','center');port_label('output',1,'CAN_Msg');
  CAN Receive (CANRX)1 : S-Function  FunctionName=CAN_Rec_P  Parameters=uint8(Module-1),uint32(ID),uint8(Frameformat-1),uint8(Newflag),uint8(FIFO),double(sampletime)  SFunctionDeploymentMode=off  EnableBusSupport=off  mask(CAN_receive){Module=CAN_2, ID=1524, Frameformat=Standard (11-bit identifier), Newflag=off, FIFO=off, sampletime=0.05}
      mask prompts: Module "CAN Port:"; ID "CAN Frame ID:"; Frameformat "CAN Frame Format:"; FIFO "Overflow flag"
      mask init:
      | maskdisplay = canrecicon(Module,ID,Frameformat,Newflag,FIFO);
      | set_param(gcb, 'MaskDisplay', maskdisplay);
      mask TypeOptions Module: CAN_0 | CAN_1 | CAN_2 | CAN_3
      mask TypeOptions Frameformat: Standard (11-bit identifier) | Extended (29-bit identifier)
      mask Display: color('blue');text(0.98,0.9,'MPC5675K','horizontalAlignment','right');color('black');text(0.5,0.6,'FlexCAN_2 Receive','horizontalAlignment','center');text(0.5,0.35,'Standard ID:1524','horizontalAlignment','center');port_label('output',1,'CAN_Msg');
  CAN Unpack1 : canmsglib/CAN Unpack  CANdbFile=D:\Work\02_LKA\LKAS\Documents\D53-SensorCAN.dbc  MsgList=Video_Lane_Next_Right_B  MsgName=Video_Lane_Next_Right_B  MsgIDType=Standard (11-bit identifier)  MsgIdentifier=1524  MsgLength=4  SignalInfo=Line_Width_5F4$17$7$2$2$1$0$1.000000e-02$0$0$1.270000e+00$#Me_Line_Changed_5F4$16$1$2$2$1$0$1$0$0$1$#TLC_5F4$8$8$2$2$1$0$1.000000e-02$0$0$2.550000e+00$#View_Range_5F4$0$8$2$2$1$0$5.000000e-01$0$0$1.275000e+02$#  NSignals=4  IDPort=off  TimestampPort=off  ErrorPort=off  RemotePort=off  LengthPort=off  StatusPort=off  StartBits=str2num('[int32(17);int32(16);int32(8);int32(0)]')  SignalSizes=str2num('[int32(7);int32(1);int32(8);int32(8)]')  ByteOrders=str2num('[int32(2);int32(2);int32(2);int32(2)]')  DataTypes=str2num('[int32(2);int32(2);int32(2);int32(2)]')  MultiplexTypes=str2num('[int32(1);int32(1);int32(1);int32(1)]')  MultiplexValues=str2num('[double(0);double(0);double(0);double(0)]')  Factors=str2num('[double(1.000000e-02);double(1);double(1.000000e-02);double(5.000000e-01)]')  Offsets=str2num('[double(0);double(0);double(0);double(0)]')  Minimums=str2num('[double(0);double(0);double(0);double(0)]')  Maximums=str2num('[double(1.270000e+00);double(1);double(2.550000e+00);double(1.275000e+02)]')  ApplyMinMax=off
      settings: SourceProductName=Simulink Real-Time  SourceProductBaseCode=XP  DataFormat=CANdb specified signals
  CAN Unpack13 : canmsglib/CAN Unpack  CANdbFile=D:\Work\02_LKA\LKAS\Documents\D53-SensorCAN.dbc  MsgList=Video_Lane_Next_Right_A  MsgName=Video_Lane_Next_Right_A  MsgIDType=Standard (11-bit identifier)  MsgIdentifier=1534  MsgLength=8  SignalInfo=C0_5FE$44$12$2$1$1$0$1.000000e-02$0$-2.048000e+01$2.047000e+01$#C1_5FE$50$10$2$1$1$0$9.765625e-04$0$-3.570000e-01$3.570000e-01$#C2_5FE$24$16$2$1$1$0$1.000000e-06$0$-3.276800e-02$3.276600e-02$#C3_5FE$8$16$2$1$1$0$4.000000e-09$0$-1.310720e-04$1.310680e-04$#Line_Type_5FE$59$3$2$2$1$0$1$0$0$7$#Quality_5FE$62$2$2$2$1$0$1$0$0$3$#  NSignals=6  IDPort=off  TimestampPort=off  ErrorPort=off  RemotePort=off  LengthPort=off  StatusPort=off  StartBits=str2num('[int32(44);int32(50);int32(24);int32(8);int32(59);int32(62)]')  SignalSizes=str2num('[int32(12);int32(10);int32(16);int32(16);int32(3);int32(2)]')  ByteOrders=str2num('[int32(2);int32(2);int32(2);int32(2);int32(2);int32(2)]')  DataTypes=str2num('[int32(1);int32(1);int32(1);int32(1);int32(2);int32(2)]')  MultiplexTypes=str2num('[int32(1);int32(1);int32(1);int32(1);int32(1);int32(1)]')  MultiplexValues=str2num('[double(0);double(0);double(0);double(0);double(0);double(0)]')  Factors=str2num('[double(1.000000e-02);double(9.765625e-04);double(1.000000e-06);double(4.000000e-09);double(1);double(1)]')  Offsets=str2num('[double(0);double(0);double(0);double(0);double(0);double(0)]')  Minimums=str2num('[double(-2.048000e+01);double(-3.570000e-01);double(-3.276800e-02);double(-1.310720e-04);double(0);double(0)]')  Maximums=str2num('[double(2.047000e+01);double(3.570000e-01);double(3.276600e-02);double(1.310680e-04);double(7);double(3)]')  ApplyMinMax=off
      settings: SourceProductName=Simulink Real-Time  SourceProductBaseCode=XP  DataFormat=CANdb specified signals
  Data Type Conversion{,6..8,10..11,14} (7 alike) : DataTypeConversion  OutDataTypeStr=single
  Data Type Conversion12 : DataTypeConversion  OutDataTypeStr=uint8
  Data Type Conversion13 : DataTypeConversion  OutDataTypeStr=uint8
  Data Type Conversion9 : DataTypeConversion  OutDataTypeStr=uint8
  Rate Transition{1..10} (10 alike) : RateTransition  Deterministic=off  OutPortSampleTime=0.01
  bsOriR1Info : Outport
  wires:
  Data Type Conversion6/1 -> Bus Creator22/3  "O_R1_C1"
  Data Type Conversion11/1 -> Bus Creator22/9  "O_R1_W"
  Data Type Conversion14/1 -> Bus Creator22/8  "O_R1_TLC"
  Data Type Conversion/1 -> Bus Creator22/4  "O_R1_C0"
  Data Type Conversion7/1 -> Bus Creator22/2  "O_R1_C2"
  Data Type Conversion9/1 -> Bus Creator22/5  "O_R1_Q"
  Data Type Conversion13/1 -> Bus Creator22/10  "O_R1_LC"
  Data Type Conversion8/1 -> Bus Creator22/1  "O_R1_C3"
  CAN Unpack13/2 -> Rate Transition2/1
  CAN Unpack13/3 -> Rate Transition3/1
  Data Type Conversion12/1 -> Bus Creator22/6  "O_R1_Type"
  Data Type Conversion10/1 -> Bus Creator22/7  "O_R1_VR"
  CAN Unpack13/1 -> Rate Transition1/1
  CAN Unpack1/4 -> Rate Transition10/1
  CAN Receive (CANRX)/1 -> CAN Unpack13/1
  CAN Unpack1/3 -> Rate Transition9/1
  CAN Unpack13/5 -> Rate Transition5/1
  CAN Unpack13/6 -> Rate Transition6/1
  CAN Unpack1/2 -> Rate Transition8/1
  CAN Unpack1/1 -> Rate Transition7/1
  CAN Unpack13/4 -> Rate Transition4/1
  Bus Creator22/1 -> bsOriR1Info/1  "bsOriR1Info"
  CAN Receive (CANRX)1/1 -> CAN Unpack1/1
  Rate Transition1/1 -> Data Type Conversion/1
  Rate Transition2/1 -> Data Type Conversion6/1
  Rate Transition3/1 -> Data Type Conversion7/1
  Rate Transition4/1 -> Data Type Conversion8/1
  Rate Transition5/1 -> Data Type Conversion12/1
  Rate Transition6/1 -> Data Type Conversion9/1
  Rate Transition7/1 -> Data Type Conversion11/1
  Rate Transition8/1 -> Data Type Conversion13/1
  Rate Transition9/1 -> Data Type Conversion14/1
  Rate Transition10/1 -> Data Type Conversion10/1
